simulink model "HindernisRegler"  (R2017a)
settings: Solver=FixedStepAuto  StartTime=0.0  StopTime=40  FixedStep=1/1000  RelTol=1e-3
values from neighbouring files (symbols this model uses):
  l_a = 0.184    [Kippreglerauslegung.m]    (also in Minv.m = 0.14; Roboterdaten.m = 0.14)
  r = 0.05    [Kippreglerauslegung.m]    (also in Minv.m; Roboterdaten.m)
libraries: simulink x3, vrlib x1
settings Model: Creator=Stephan  LastModifiedBy=Timo

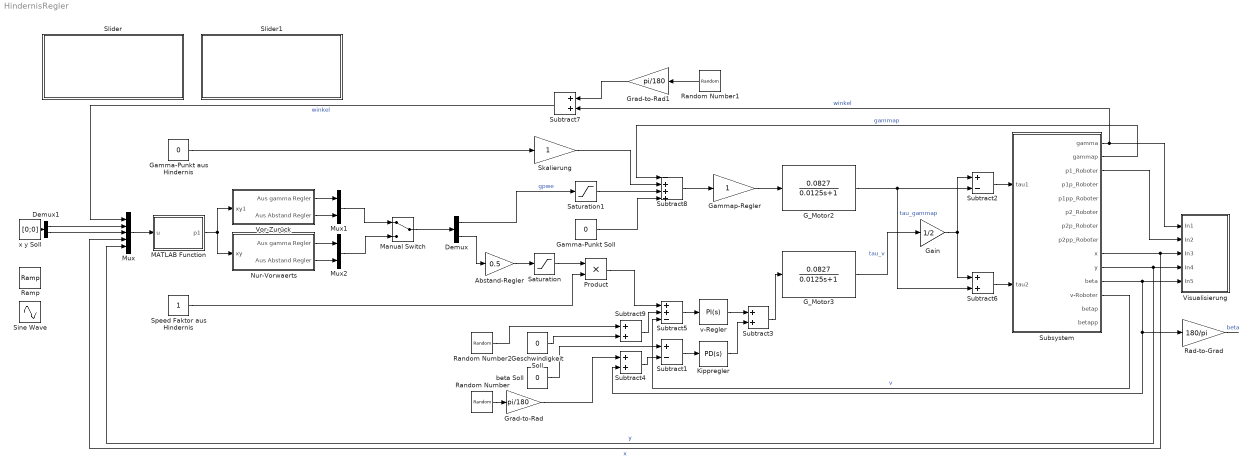
== system HindernisRegler ==
  "Abstand-Regler " : Gain  Gain=0.5
  Demux : Demux  Outputs=2
  Demux1 : Demux  Outputs=2
  G_Motor2 : TransferFcn  Numerator=0.0827  Denominator=[0.0125 1]
  G_Motor3 : TransferFcn  Numerator=0.0827  Denominator=[0.0125 1]
  Gain : Gain  Gain=1/2
  Gamma-Punkt Soll : Constant  Value=0
  Gamma-Punkt aus Hindernis : Constant  Value=0
  Gammap-Regler : Gain
  Geschwindigkeit Soll : Constant  Value=0
  Grad-to-Rad : Gain  Gain=pi/180
  Grad-to-Rad1 : Gain  Gain=pi/180
  Kippregler : simulink/Continuous/PID Controller  Controller=PD  TimeDomain=Continuous-time  SampleTime=-1  IntegratorMethod=Forward Euler  FilterMethod=Forward Euler  Form=Parallel  UseFilter=on  ControllerParametersSource=internal  P=-60  I=0  D=-4.27  N=1000  InitialConditionSource=internal  InitialConditionForIntegrator=0  InitialConditionForFilter=0  ExternalReset=none  LimitOutput=off  UpperSaturationLimit=inf  LowerSaturationLimit=-inf  LinearizeAsGain=on  AntiWindupMode=none  Kb=1  TrackingMode=off  Kt=1  PParamMin=[]  PParamMax=[]  IParamMin=[]  IParamMax=[]  DParamMin=[]  DParamMax=[]  NParamMin=[]  NParamMax=[]  KbParamMin=[]  KbParamMax=[]  KtParamMin=[]  KtParamMax=[]  POutMin=[]  POutMax=[]  IOutMin=[]  IOutMax=[]  DOutMin=[]  DOutMax=[]  NOutMin=[]  NOutMax=[]  KbOutMin=[]  KbOutMax=[]  KtOutMin=[]  KtOutMax=[]  IntegratorOutMin=[]  IntegratorOutMax=[]  FilterOutMin=[]  FilterOutMax=[]  SumOutMin=[]  SumOutMax=[]  SumI1OutMin=[]  SumI1OutMax=[]  SumI2OutMin=[]  SumI2OutMax=[]  SumI3OutMin=[]  SumI3OutMax=[]  SumDOutMin=[]  SumDOutMax=[]  SaturationOutMin=[]  SaturationOutMax=[]  IntegratorContinuousStateAttributes=''  IntegratorStateMustResolveToSignalObject=off  IntegratorRTWStateStorageClass=Auto  FilterContinuousStateAttributes=''  FilterStateMustResolveToSignalObject=off  FilterRTWStateStorageClass=Auto  DifferentiatorICPrevScaledInput=0  DifferentiatorOutMin=[]  DifferentiatorOutMax=[]  InitialConditionSetting=State (most efficient)
  MATLAB Function : MATLAB Function  TreatAsAtomicUnit=on
  Manual Switch : ManualSwitch
  Mux : Mux  Inputs=5
  Mux1 : Mux  Inputs=2
  Mux2 : Mux  Inputs=2
  Nur-Vorwaerts : Subsystem
  Product : Product
  Rad-to-Grad : Gain  Gain=180/pi
  Ramp : simulink/Sources/Ramp  slope=0.2  start=0  X0=0
  Random Number : RandomNumber  Mean=0.5  SampleTime=0.01
  Random Number1 : RandomNumber  Variance=2  SampleTime=0.01
  Random Number2 : RandomNumber  Variance=0.001  SampleTime=0.01
  Saturation : Saturate
  Saturation1 : Saturate  UpperLimit=3  LowerLimit=-3
  Sine Wave : Sin  SampleTime=0
  Skalierung : Gain
  Slider : Subsystem  DialogController=hmiCreateDDGDialog  IsWebBlock=on  mask(MWDashboardBlock){webBlockId=772f47d9-01a1-4a0e-b5ee-e24562c78f27, webBlockType=slider, ShowInLibBrowser=on, ShowInitialText=on, HMISrcModelName=HindernisRegler}
      mask prompts: webBlockId "WebBlock Id"; webBlockType "WebBlock Type"; HMISrcModelName "Source Model"
      mask help: SimulinkHMI:dialogs:SliderDialogDesc
      mask Help: helpview([docroot '/mapfiles/simulink.map'], 'hmi_slider')
      mask Display:
      | if strcmp(get_param(bdroot(gcb),'BlockDiagramType'), 'library')
      |     image([(matlabroot) '/toolbox/simulink/hmi/icons/Slider.png']);
      | end
  Slider1 : Subsystem  DialogController=hmiCreateDDGDialog  IsWebBlock=on  mask(MWDashboardBlock){webBlockId=0b4e93f3-1b2a-484e-ac47-cdbb2b4f16cb, webBlockType=slider, ShowInLibBrowser=on, ShowInitialText=on, HMISrcModelName=HindernisRegler}
      mask prompts: webBlockId "WebBlock Id"; webBlockType "WebBlock Type"; HMISrcModelName "Source Model"
      mask help: SimulinkHMI:dialogs:SliderDialogDesc
      mask Help: helpview([docroot '/mapfiles/simulink.map'], 'hmi_slider')
      mask Display:
      | if strcmp(get_param(bdroot(gcb),'BlockDiagramType'), 'library')
      |     image([(matlabroot) '/toolbox/simulink/hmi/icons/Slider.png']);
      | end
  Speed Faktor aus Hindernis : Constant
  Subsystem : Subsystem
  Subtract1 : Sum  Inputs=+-
  Subtract2 : Sum  Inputs=+-
  Subtract{3..4,6..7,9} (5 alike) : Sum
  Subtract5 : Sum  Inputs=++-
  Subtract8 : Sum  Inputs=-+++
  Visualisierung : Subsystem
  Vor-Zurück : Subsystem
  beta Soll : Constant  Value=0
  v-Regler : simulink/Continuous/PID Controller  Controller=PI  TimeDomain=Continuous-time  SampleTime=-1  IntegratorMethod=Forward Euler  FilterMethod=Forward Euler  Form=Parallel  UseFilter=on  ControllerParametersSource=internal  P=-4.5  I=-1.69  D=0.003  N=1000  InitialConditionSource=internal  InitialConditionForIntegrator=0  InitialConditionForFilter=0  ExternalReset=none  LimitOutput=off  UpperSaturationLimit=inf  LowerSaturationLimit=-inf  LinearizeAsGain=on  AntiWindupMode=none  Kb=1  TrackingMode=off  Kt=1  PParamMin=[]  PParamMax=[]  IParamMin=[]  IParamMax=[]  DParamMin=[]  DParamMax=[]  NParamMin=[]  NParamMax=[]  KbParamMin=[]  KbParamMax=[]  KtParamMin=[]  KtParamMax=[]  POutMin=[]  POutMax=[]  IOutMin=[]  IOutMax=[]  DOutMin=[]  DOutMax=[]  NOutMin=[]  NOutMax=[]  KbOutMin=[]  KbOutMax=[]  KtOutMin=[]  KtOutMax=[]  IntegratorOutMin=[]  IntegratorOutMax=[]  FilterOutMin=[]  FilterOutMax=[]  SumOutMin=[]  SumOutMax=[]  SumI1OutMin=[]  SumI1OutMax=[]  SumI2OutMin=[]  SumI2OutMax=[]  SumI3OutMin=[]  SumI3OutMax=[]  SumDOutMin=[]  SumDOutMax=[]  SaturationOutMin=[]  SaturationOutMax=[]  IntegratorContinuousStateAttributes=''  IntegratorStateMustResolveToSignalObject=off  IntegratorRTWStateStorageClass=Auto  FilterContinuousStateAttributes=''  FilterStateMustResolveToSignalObject=off  FilterRTWStateStorageClass=Auto  DifferentiatorICPrevScaledInput=0  DifferentiatorOutMin=[]  DifferentiatorOutMax=[]  InitialConditionSetting=State (most efficient)
  x y Soll : Constant  Value=[0;0]
  wires:
  Subsystem/11(beta) -> Subtract4/2, Rad-to-Grad/1, Visualisierung/5(In5)
  Gammap-Regler/1 -> G_Motor2/1
  Subsystem/2(gammap) -> Subtract8/1  "gammap"
  Gamma-Punkt Soll/1 -> Subtract8/4
  Gain/1 -> Subtract6/1, Subtract2/1
  G_Motor3/1 -> Gain/1  "tau_v"
  Subtract6/1 -> Subsystem/2(tau2)
  G_Motor2/1 -> Subtract2/2, Subtract6/2  "tau_gammap"
  Subtract2/1 -> Subsystem/1(tau1)
  Subtract1/1 -> Kippregler/1
  beta Soll/1 -> Subtract1/1
  Subtract8/1 -> Gammap-Regler/1
  Subsystem/12(v-Roboter) -> Subtract5/3  "v"
  Subsystem/3(p1_Roboter) -> Visualisierung/2(In2)
  Subtract5/1 -> v-Regler/1
  Subtract3/1 -> G_Motor3/1
  Kippregler/1 -> Subtract3/2
  Rad-to-Grad/1 -> ?  "beta"
  Random Number/1 -> Grad-to-Rad/1
  Subtract4/1 -> Subtract1/2
  Grad-to-Rad/1 -> Subtract4/1
  v-Regler/1 -> Subtract3/1
  Subtract9/1 -> Subtract5/2
  Subtract7/1 -> Mux/1  "winkel"
  Subsystem/10(y) -> Mux/5, Visualisierung/4(In4)  "y"
  Subsystem/9(x) -> Mux/4, Visualisierung/3(In3)  "x"
  x y Soll/1 -> Demux1/1
  "Abstand-Regler "/1 -> Saturation/1
  Mux/1 -> MATLAB Function/1(u)
  MATLAB Function/1(p1) -> Vor-Zurück/1(xy1), Nur-Vorwaerts/1(xy)
  Saturation/1 -> Product/1
  Demux/1 -> Saturation1/1  "gpwe"
  Demux/2 -> "Abstand-Regler "/1
  Manual Switch/1 -> Demux/1
  Mux2/1 -> Manual Switch/2
  Nur-Vorwaerts/2(Aus Abstand Regler) -> Mux2/2
  Nur-Vorwaerts/1(Aus gamma Regler) -> Mux2/1
  Vor-Zurück/2(Aus Abstand Regler) -> Mux1/2
  Vor-Zurück/1(Aus gamma Regler) -> Mux1/1
  Mux1/1 -> Manual Switch/1
  Saturation1/1 -> Subtract8/3
  Random Number1/1 -> Grad-to-Rad1/1
  Subsystem/1(gamma) -> Subtract7/2, Visualisierung/1(In1)  "winkel"
  Grad-to-Rad1/1 -> Subtract7/1
  Geschwindigkeit Soll/1 -> Subtract9/2
  Random Number2/1 -> Subtract9/1
  Demux1/2 -> Mux/3
  Demux1/1 -> Mux/2
  Gamma-Punkt aus Hindernis/1 -> Skalierung/1
  Skalierung/1 -> Subtract8/2
  Product/1 -> Subtract5/1
  Speed Faktor aus Hindernis/1 -> Product/2

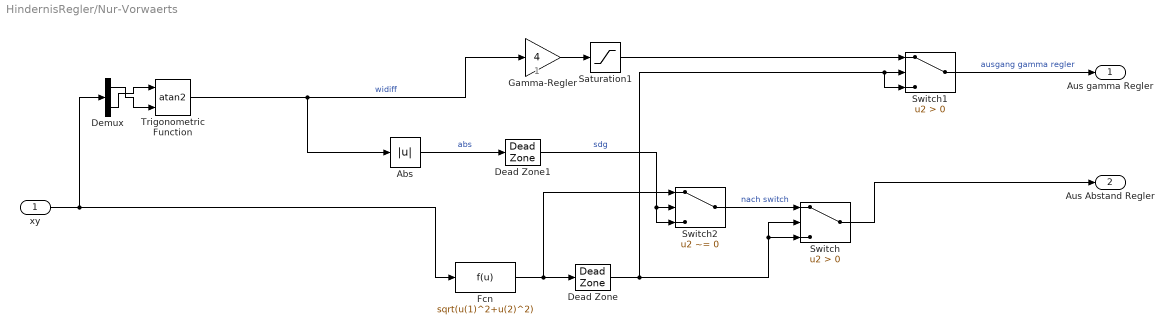
== system HindernisRegler/Nur-Vorwaerts ==
  note: 1
  xy : Inport
  Abs : Abs
  Dead Zone : DeadZone  LowerValue=-0.05  UpperValue=0.05  SaturateOnIntegerOverflow=on
  Dead Zone1 : DeadZone  LowerValue=2.96  UpperValue=2*pi
  Demux : Demux  Outputs=2
  Fcn : Fcn  Expr=sqrt(u(1)^2+u(2)^2)
  Gamma-Regler : Gain  Gain=4
  Saturation1 : Saturate  UpperLimit=3  LowerLimit=-3
  Switch : Switch  Criteria=u2 > Threshold
  Switch1 : Switch  Criteria=u2 > Threshold
  Switch2 : Switch  Criteria=u2 ~= 0
  Trigonometric Function : Trigonometry  Operator=atan2
  Aus gamma Regler : Outport
  Aus Abstand Regler : Outport  Port=2
  wires:
  Abs/1 -> Dead Zone1/1  "abs"
  xy/1 -> Demux/1, Fcn/1
  Dead Zone1/1 -> Switch2/3, Switch2/2  "sdg"
  Switch2/1 -> Switch/1  "nach switch"
  Saturation1/1 -> Switch1/1
  Switch1/1 -> Aus gamma Regler/1  "ausgang gamma regler"
  Gamma-Regler/1 -> Saturation1/1
  Demux/1 -> Trigonometric Function/2
  Demux/2 -> Trigonometric Function/1
  Trigonometric Function/1 -> Abs/1, Gamma-Regler/1  "widiff"
  Dead Zone/1 -> Switch1/3, Switch1/2, Switch/2, Switch/3
  Fcn/1 -> Switch2/1, Dead Zone/1
  Switch/1 -> Aus Abstand Regler/1

== system HindernisRegler/Slider ==

== system HindernisRegler/Slider1 ==

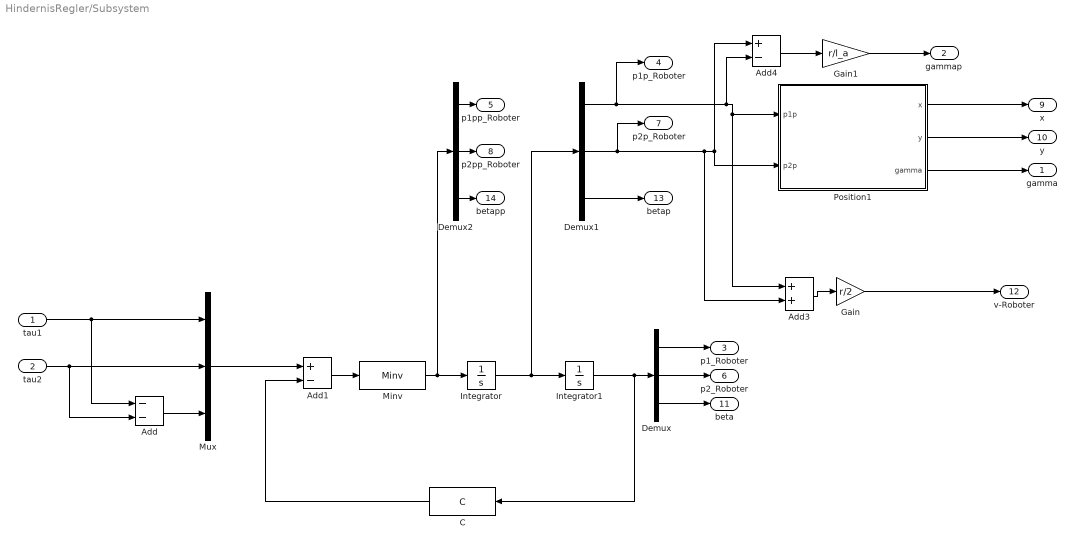
== system HindernisRegler/Subsystem ==
  tau1 : Inport
  tau2 : Inport  Port=2
  Add : Sum  Inputs=--
  Add1 : Sum  Inputs=+-
  Add3 : Sum
  Add4 : Sum  Inputs=+-
  C : MATLABFcn  MATLABFcn=C  OutputDimensions=3
  Demux : Demux  Outputs=3
  Demux1 : Demux  Outputs=3
  Demux2 : Demux  Outputs=3
  Gain : Gain  Gain=r/2
  Gain1 : Gain  Gain=r/l_a
  Integrator : Integrator
  Integrator1 : Integrator
  Minv : MATLABFcn  MATLABFcn=Minv  OutputDimensions=3
  Mux : Mux  Inputs=3
  Position1 : Subsystem
  gamma : Outport
  gammap : Outport  Port=2
  p1_Roboter : Outport  Port=3
  p1p_Roboter : Outport  Port=4
  p1pp_Roboter : Outport  Port=5
  p2_Roboter : Outport  Port=6
  p2p_Roboter : Outport  Port=7
  p2pp_Roboter : Outport  Port=8
  x : Outport  Port=9
  y : Outport  Port=10
  beta : Outport  Port=11
  v-Roboter : Outport  Port=12
  betap : Outport  Port=13
  betapp : Outport  Port=14
  wires:
  tau1/1 -> Mux/1, Add/1
  tau2/1 -> Mux/2, Add/2
  Add/1 -> Mux/3
  Mux/1 -> Add1/1
  Integrator/1 -> Demux1/1, Integrator1/1
  Add1/1 -> Minv/1
  Integrator1/1 -> C/1, Demux/1
  Demux/1 -> p1_Roboter/1
  Demux/2 -> p2_Roboter/1
  Demux/3 -> beta/1
  Demux1/3 -> betap/1
  Demux1/2 -> p2p_Roboter/1, Add4/1, Position1/2(p2p), Add3/2
  Demux1/1 -> p1p_Roboter/1, Add4/2, Position1/1(p1p), Add3/1
  C/1 -> Add1/2
  Demux2/2 -> p2pp_Roboter/1
  Demux2/1 -> p1pp_Roboter/1
  Demux2/3 -> betapp/1
  Minv/1 -> Demux2/1, Integrator/1
  Add3/1 -> Gain/1
  Add4/1 -> Gain1/1
  Gain1/1 -> gammap/1
  Gain/1 -> v-Roboter/1
  Position1/1(x) -> x/1
  Position1/2(y) -> y/1
  Position1/3(gamma) -> gamma/1

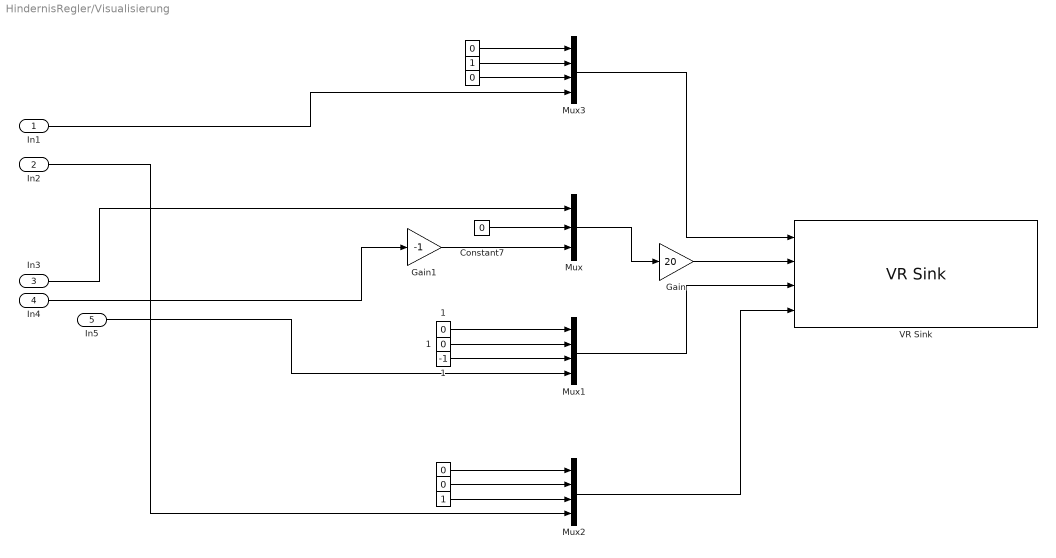
== system HindernisRegler/Visualisierung ==
  In1 : Inport
  In2 : Inport  Port=2
  In3 : Inport  Port=3
  In4 : Inport  Port=4
  In5 : Inport  Port=5
  "   " : Constant  Value=0
  "     " : Constant  Value=0
  "      " : Constant
  "               " : Constant  Value=0
  "                       " : Constant
  "                                " : Constant  Value=0
  "      1" : Constant  Value=-1
  "     1" : Constant  Value=0
  "   1" : Constant  Value=0
  Constant7 : Constant  Value=0
  Gain : Gain  Gain=20
  Gain1 : Gain  Gain=-1
  Mux : Mux  Inputs=3
  Mux1 : Mux
  Mux2 : Mux
  Mux3 : Mux
  VR Sink : vrlib/VR Sink  InstantiateOnLoad=on  SampleTime=0.1  ViewEnable=on  RemoteChange=off  RemoteView=off  FieldsWritten=SegwayPosition.rotation.4.1.1.double#SegwayPosition.translation.3.1.1.double#SegwayKippwinkel.rotation.4.1.1.double#Radmarkierungen.rotation.4.1.1.double  WorldFileName=SegwayWorldModell.wrl  WorldDescription=Straight Road Strip - 2 Lanes  AutoView=off  VideoDimensions=[]  AllowVariableSize=off  FigureProperties="{'Position', 'Name', 'Viewpoint', 'CameraBound', 'CameraDirection', 'CameraPosition', 'CameraUpVector', 'ZoomFactor', 'Antialiasing', 'Headlight', 'Lighting', 'NavPanel', 'Sound', 'StatusBar', 'Stereo3D', 'Stereo3DCameraOffset', 'Stereo3DHIT', 'ToolBar', 'Textures', 'Transparency', 'Triad', 'Wireframe', 'NavZones', 'NavMode', 'NavSpeed', 'CaptureFileFormat', 'CaptureFileName', 'Record2DCompressMethod', 'Record2DCompressQuality', 'Record2D', 'Record2DFileName', 'Record2DFPS'; [9.6200000000000000e+02   8.4000000000000000e+01   9.5800000000000000e+02   9.0400000000000000e+02], 'Straight Road Strip - 2 Lanes', 'Observe Car at Start', 'on', [0.0000000000000000e+00   0.0000000000000000e+00  -1.0000000000000000e+00], [0.0000000000000000e+00   0.0000000000000000e+00   2.9000000000000000e+01], [0.0000000000000000e+00   1.0000000000000000e+00   0.0000000000000000e+00], [1.0000000000000000e+00], 'on', 'off', 'on', 'halfbar', 'on', 'on', 'off', [1.0000000149011612e-01], [0.0000000000000000e+00], 'on', 'on', 'on', 'none', 'off', 'off', 'walk', 'normal', 'tif', '%f_anim_%n.tif', 'auto', [7.5000000000000000e+01], 'off', '%f_anim_%n.avi', 'auto'}"
      settings: SourceProductBaseCode=VR
  wires:
  In3/1 -> Mux/1
  "     1"/1 -> Mux1/2
  "                       "/1 -> Mux3/2
  "   1"/1 -> Mux1/1
  "   "/1 -> Mux2/1
  In2/1 -> Mux2/4
  "      "/1 -> Mux2/3
  "               "/1 -> Mux3/3
  Mux1/1 -> VR Sink/3
  Mux2/1 -> VR Sink/4
  In1/1 -> Mux3/4
  "                                "/1 -> Mux3/1
  "      1"/1 -> Mux1/3
  Constant7/1 -> Mux/2
  In4/1 -> Gain1/1
  Mux3/1 -> VR Sink/1
  "     "/1 -> Mux2/2
  Mux/1 -> Gain/1
  In5/1 -> Mux1/4
  Gain/1 -> VR Sink/2
  Gain1/1 -> Mux/3

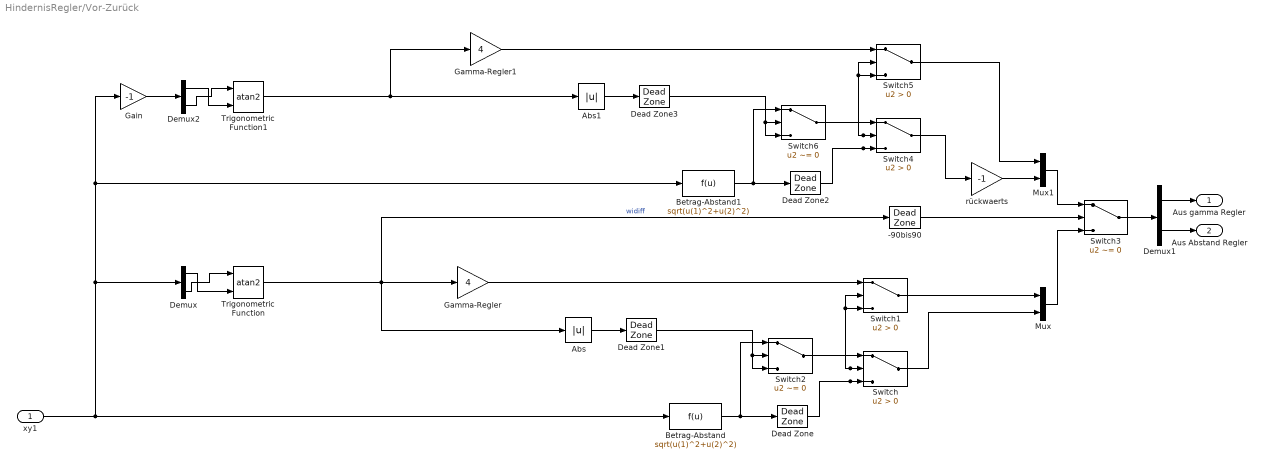
== system HindernisRegler/Vor-Zurück ==
  xy1 : Inport
  -90bis90 : DeadZone  LowerValue=-pi/2  UpperValue=pi/2
  Abs : Abs
  Abs1 : Abs
  Betrag-Abstand : Fcn  Expr=sqrt(u(1)^2+u(2)^2)
  Betrag-Abstand1 : Fcn  Expr=sqrt(u(1)^2+u(2)^2)
  Dead Zone : DeadZone  LowerValue=-0.05  UpperValue=0.05  SaturateOnIntegerOverflow=on
  Dead Zone1 : DeadZone  LowerValue=(pi/2)-0.15  UpperValue=2*pi
  Dead Zone2 : DeadZone  LowerValue=-0.05  UpperValue=0.05  SaturateOnIntegerOverflow=on
  Dead Zone3 : DeadZone  LowerValue=(pi/2)-0.15  UpperValue=2*pi
  Demux : Demux  Outputs=2
  Demux1 : Demux  Outputs=2
  Demux2 : Demux  Outputs=2
  Gain : Gain  Gain=-1
  Gamma-Regler : Gain  Gain=4
  Gamma-Regler1 : Gain  Gain=4
  Mux : Mux  Inputs=2
  Mux1 : Mux  Inputs=2
  Switch{,1,4..5} (4 alike) : Switch  Criteria=u2 > Threshold
  Switch2 : Switch  Criteria=u2 ~= 0
  Switch3 : Switch  Criteria=u2 ~= 0
  Switch6 : Switch  Criteria=u2 ~= 0
  Trigonometric Function : Trigonometry  Operator=atan2
  Trigonometric Function1 : Trigonometry  Operator=atan2
  rückwaerts : Gain  Gain=-1
  Aus gamma Regler : Outport
  Aus Abstand Regler : Outport  Port=2
  wires:
  Abs/1 -> Dead Zone1/1
  xy1/1 -> Betrag-Abstand1/1, Gain/1, Demux/1, Betrag-Abstand/1
  Dead Zone1/1 -> Switch2/3, Switch2/2
  Switch2/1 -> Switch/1
  Switch1/1 -> Mux/1
  Demux/1 -> Trigonometric Function/2
  Demux/2 -> Trigonometric Function/1
  Dead Zone/1 -> Switch1/2, Switch1/3, Switch/2, Switch/3
  Betrag-Abstand/1 -> Switch2/1, Dead Zone/1
  Switch/1 -> Mux/2
  -90bis90/1 -> Switch3/2
  Gamma-Regler/1 -> Switch1/1
  Demux1/2 -> Aus Abstand Regler/1
  Demux1/1 -> Aus gamma Regler/1
  Switch3/1 -> Demux1/1
  Mux/1 -> Switch3/3
  Demux2/2 -> Trigonometric Function1/1
  Gain/1 -> Demux2/1
  Demux2/1 -> Trigonometric Function1/2
  Mux1/1 -> Switch3/1
  Switch4/1 -> rückwaerts/1
  Gamma-Regler1/1 -> Switch5/1
  Dead Zone3/1 -> Switch6/3, Switch6/2
  Betrag-Abstand1/1 -> Switch6/1, Dead Zone2/1
  Dead Zone2/1 -> Switch5/2, Switch5/3, Switch4/2, Switch4/3
  Switch6/1 -> Switch4/1
  Abs1/1 -> Dead Zone3/1
  Switch5/1 -> Mux1/1
  Trigonometric Function1/1 -> Gamma-Regler1/1, Abs1/1
  rückwaerts/1 -> Mux1/2
  Trigonometric Function/1 -> -90bis90/1, Gamma-Regler/1, Abs/1  "widiff"

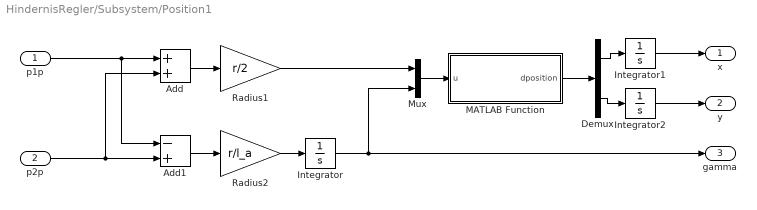
== system HindernisRegler/Subsystem/Position1 ==
  p1p : Inport
  p2p : Inport  Port=2
  Add : Sum
  Add1 : Sum  Inputs=-+
  Demux : Demux  Outputs=2
  Integrator : Integrator
  Integrator1 : Integrator
  Integrator2 : Integrator
  MATLAB Function : MATLAB Function  TreatAsAtomicUnit=on
  Mux : Mux  Inputs=2
  Radius1 : Gain  Gain=r/2
  Radius2 : Gain  Gain=r/l_a
  x : Outport
  y : Outport  Port=2
  gamma : Outport  Port=3
  wires:
  Add/1 -> Radius1/1
  p2p/1 -> Add/2, Add1/2
  Add1/1 -> Radius2/1
  p1p/1 -> Add1/1, Add/1
  Integrator/1 -> gamma/1, Mux/2
  Radius2/1 -> Integrator/1
  MATLAB Function/1(dposition) -> Demux/1
  Demux/1 -> Integrator1/1
  Integrator1/1 -> x/1
  Demux/2 -> Integrator2/1
  Integrator2/1 -> y/1
  Radius1/1 -> Mux/1
  Mux/1 -> MATLAB Function/1(u)

== matlab function HindernisRegler/MATLAB Function ==
  data: u input; p1 output
function p1 = fcn(u)
%u(1) gamma
%u(2) x soll
%u(3) y soll
%u(4) x
%u(5) y

T10 = [ cos(u(1)), sin(u(1)) ; -sin(u(1)), cos(u(1))];

p1 = T10*([u(2); u(3)] - [u(4); u(5)]);

== matlab function HindernisRegler/Subsystem/Position1/MATLAB Function ==
  data: u input; dposition output
function dposition  = fcn(u)

dx = u(1);
gamma = u(2);

dposition = dx*[cos(gamma); sin(gamma)];
